simulink model "project_2023_11_27_p68"  (R2017b)
settings: Solver=VariableStepAuto  StartTime=0.0  StopTime=100  RelTol=1e-3
settings Model: Creator=Administrator  LastModifiedBy=Administrator

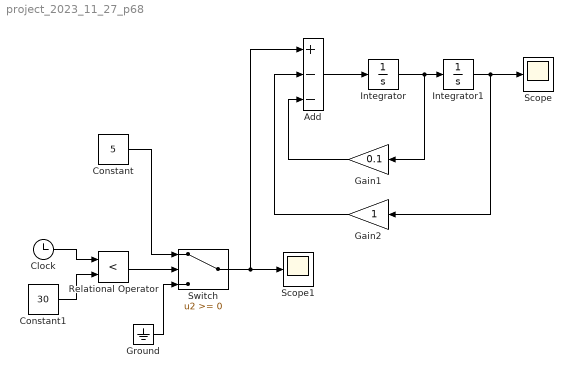
== system project_2023_11_27_p68 ==
  Add : Sum  Inputs=+--
  Clock : Clock
  Constant : Constant  Value=5
  Constant1 : Constant  Value=30
  Gain1 : Gain  Gain=0.1
  Gain2 : Gain
  Ground : Ground
  Integrator : Integrator
  Integrator1 : Integrator
  Relational Operator : RelationalOperator  Operator=<  OutDataTypeStr=boolean  RndMeth=Simplest
  Scope : Scope
  Scope1 : Scope
  Switch : Switch
  wires:
  Integrator1/1 -> Gain2/1, Scope/1
  Integrator/1 -> Gain1/1, Integrator1/1
  Add/1 -> Integrator/1
  Gain1/1 -> Add/3
  Gain2/1 -> Add/2
  Clock/1 -> Relational Operator/1
  Constant1/1 -> Relational Operator/2
  Relational Operator/1 -> Switch/2
  Ground/1 -> Switch/3
  Constant/1 -> Switch/1
  Switch/1 -> Add/1, Scope1/1
